simulink model "pendulum"  (Simulink 8.5)
settings: Solver=ode45  StartTime=0.0  StopTime=10  RelTol=1e-3
libraries: vrlib x2
settings Model: Creator=Abdre  LastModifiedBy=Abdre
settings DataIOCC: SignalLoggingSaveFormat=Dataset
settings OptimizationCC: ExpressionDepthLimit=128
settings DebuggingCC: UnderspecifiedInitializationDetection=Simplified  MergeDetectMultiDrivingBlocksExec=error  FcnCallInpInsideContextMsg=EnableAllAsError  StateNameClashWarn=none
settings GRTTargetCC: CombineOutputUpdateFcns=on  GRTInterface=off

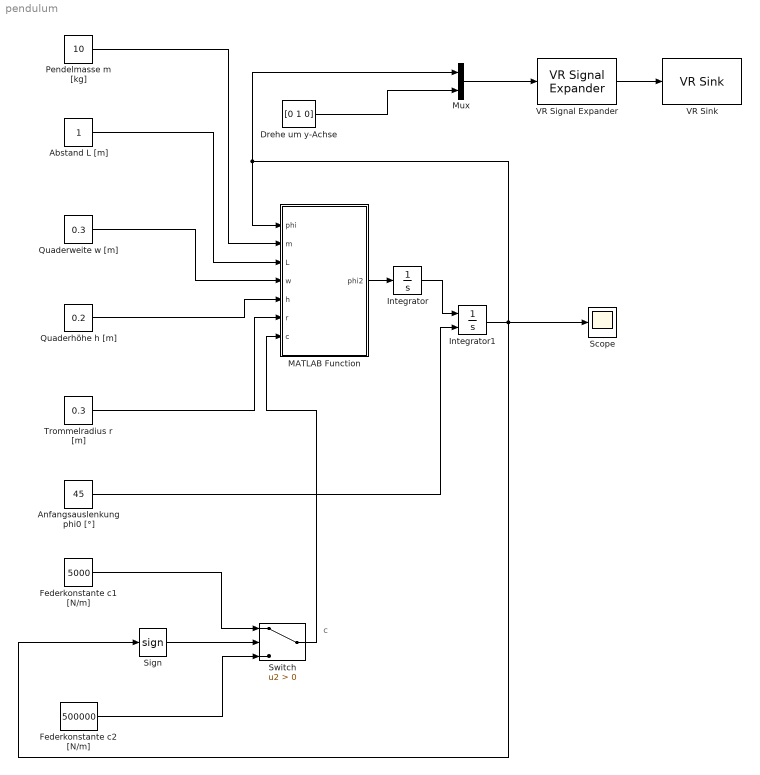
== system pendulum ==
  note: c
  Abstand L [m] : Constant
  Anfangsauslenkung phi0 [°] : Constant  Value=45
  Drehe um y-Achse : Constant  Value=[0 1 0]
  Federkonstante c1 [N/m] : Constant  Value=5000
  Federkonstante c2 [N/m] : Constant  Value=500000
  Integrator : Integrator
  Integrator1 : Integrator  InitialConditionSource=external
  MATLAB Function : MATLAB Function  TreatAsAtomicUnit=on
  Mux : Mux  Inputs=2
  Pendelmasse m [kg] : Constant  Value=10
  Quaderhöhe h [m] : Constant  Value=0.2
  Quaderweite w [m] : Constant  Value=0.3
  Scope : Scope
  Sign : Signum
  Switch : Switch  Criteria=u2 > Threshold
  Trommelradius r [m] : Constant  Value=0.3
  VR Signal Expander : vrlib/VR Signal Expander  outwidth=4  outidx=[4 1 2 3]
  VR Sink : vrlib/VR Sink  InstantiateOnLoad=on  SampleTime=0.005  ViewEnable=on  RemoteChange=off  RemoteView=off  FieldsWritten=Seiltrommel.rotation.4.1.1.double  WorldFileName=CrazyPendlm.wrl  AutoView=off  VideoDimensions=[]  AllowVariableSize=off
  wires:
  Federkonstante c1 [N/m]/1 -> Switch/1
  Federkonstante c2 [N/m]/1 -> Switch/3
  Switch/1 -> MATLAB Function/7(c)
  Sign/1 -> Switch/2
  MATLAB Function/1(phi2) -> Integrator/1
  Integrator/1 -> Integrator1/1
  Integrator1/1 -> MATLAB Function/1(phi), Mux/1, Scope/1, Sign/1
  Abstand L [m]/1 -> MATLAB Function/3(L)
  Quaderweite w [m]/1 -> MATLAB Function/4(w)
  Pendelmasse m [kg]/1 -> MATLAB Function/2(m)
  Quaderhöhe h [m]/1 -> MATLAB Function/5(h)
  Trommelradius r [m]/1 -> MATLAB Function/6(r)
  Anfangsauslenkung phi0 [°]/1 -> Integrator1/2
  Mux/1 -> VR Signal Expander/1
  Drehe um y-Achse/1 -> Mux/2
  VR Signal Expander/1 -> VR Sink/1

== matlab function MATLAB Function ==
  data: phi input double; m input double; L input double; w input double; h input double; r input double; c input double; phi2 output double
function phi2 = fcn(phi,m,L,w,h,r,c)
phiBog = phi * pi/180;
phi2 = (-c*2*pi*r^2*cos(phiBog)*(phi/360))/((1/12)*m*(w^2+h^2)+m*(L+(h/2))^2);
